simulink model "SRT_ECU_1"  (R2014a)
settings: Solver=FixedStepDiscrete  StartTime=0.0  StopTime=10.0  FixedStep=0.0005  RelTol=1e-3
libraries: ec55xxlib x10
settings Model: Creator=liuencheng  LastModifiedBy=liuencheng
settings OptimizationCC: InlineParams=on  InlineInvariantSignals=on  RollThreshold=9  StateBitsets=on  DataBitsets=on  UseTempVars=on  ZeroExternalMemoryAtStartup=off  ZeroInternalMemoryAtStartup=off  EfficientFloat2IntCast=on  OptimizeModelRefInitCode=on  LifeSpan=1
settings DebuggingCC: InheritedTsInSrcMsg=none
settings HardwareCC: ProdLargestAtomicInteger=Long  ProdLargestAtomicFloat=Double  ProdIntDivRoundTo=Zero  ProdEndianess=BigEndian  ProdHWDeviceType=Freescale MPC5500
settings RTWCC: SystemTargetFile=ec55xx.tlc  MakeCommand=make_rtw optimized_fixed_point=1  GenerateMakefile=off  TemplateMakefile=ec55xx_lcc.tmf  Description=Target for EC55XX  GenerateReport=on  ProcessScript=ec55xx_make_rtw_hook  IncludeHyperlinkInReport=on  LaunchReport=on
settings CodeAppCC: IgnoreCustomStorageClasses=off
settings STFCustomTargetCC: ModelReferenceCompliant=off  ConcurrentExecutionCompliant=off  IncludeMdlTerminateFcn=off  GeneratePreprocessorConditionals=Use local settings  CombineOutputUpdateFcns=on  SuppressErrorStatus=on  ERTCustomFileBanners=on  SupportContinuousTime=off  SupportNonInlinedSFcns=off  MATLABClassNameForMDSCustomization=Simulink.SoftwareTarget.ERTCustomization  GRTInterface=off  SystemTargetFile=ec55xx.tlc
settings ERTTargetCC: GenerateSampleERTMain=off  ModelReferenceCompliant=off  IncludeMdlTerminateFcn=off  SuppressErrorStatus=on  GenerateASAP2=on  ERTSrcFileBannerTemplate=ec55xx_code_template.cgt  ERTHdrFileBannerTemplate=ec55xx_code_template.cgt  ERTDataSrcFileTemplate=ec55xx_code_template.cgt  ERTDataHdrFileTemplate=ec55xx_code_template.cgt  ERTCustomFileTemplate=ec55xx_file_process.tlc

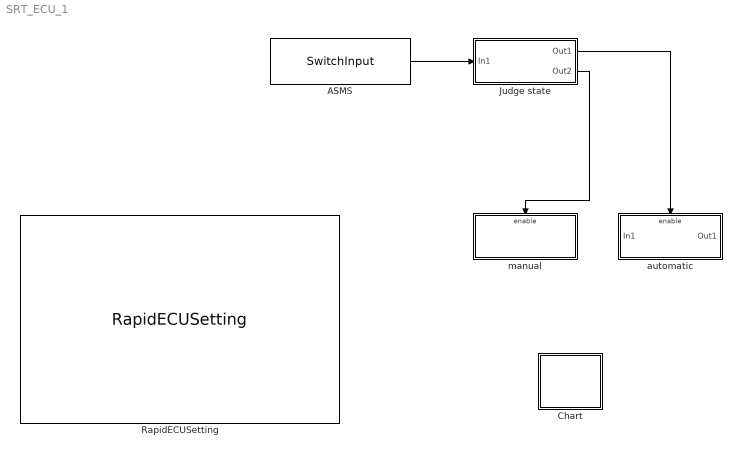
== system SRT_ECU_1 ==
  ASMS : ec55xxlib/RapidECU_U1/01SwitchInput/SwitchInput  channel=26: I_SW07_L  sampletime=-1
  Chart : Stateflow chart  TreatAsAtomicUnit=on
  Judge state : Subsystem
  RapidECUSetting : ec55xxlib/RapidECU_U2/RapidECUSetting
      link override RTI: rtiperiod=0.0005
  automatic : Subsystem  TreatAsAtomicUnit=on
  manual : Subsystem  TreatAsAtomicUnit=on
  wires:
  ASMS/1 -> Judge state/1(In1)
  Judge state/1(Out1) -> automatic/Enable
  Judge state/2(Out2) -> manual/Enable

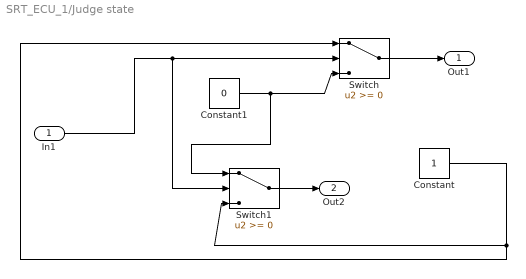
== system SRT_ECU_1/Judge state ==
  In1 : Inport
  Constant : Constant
  Constant1 : Constant  Value=0
  Switch : Switch
  Switch1 : Switch
  Out1 : Outport
  Out2 : Outport  Port=2
  wires:
  Switch/1 -> Out1/1
  Constant/1 -> Switch/1, Switch1/3
  Constant1/1 -> Switch1/1, Switch/3
  Switch1/1 -> Out2/1
  In1/1 -> Switch1/2, Switch/2

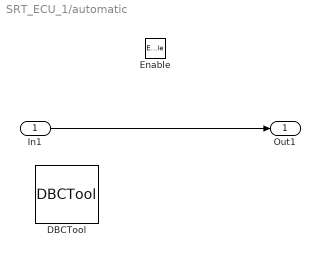
== system SRT_ECU_1/automatic ==
  In1 : Inport
  Enable : EnablePort
  DBCTool : ec55xxlib/RapidECU_U1/12DBCTool/DBCTool  dbcenable=off
  Out1 : Outport
  wires:
  In1/1 -> Out1/1

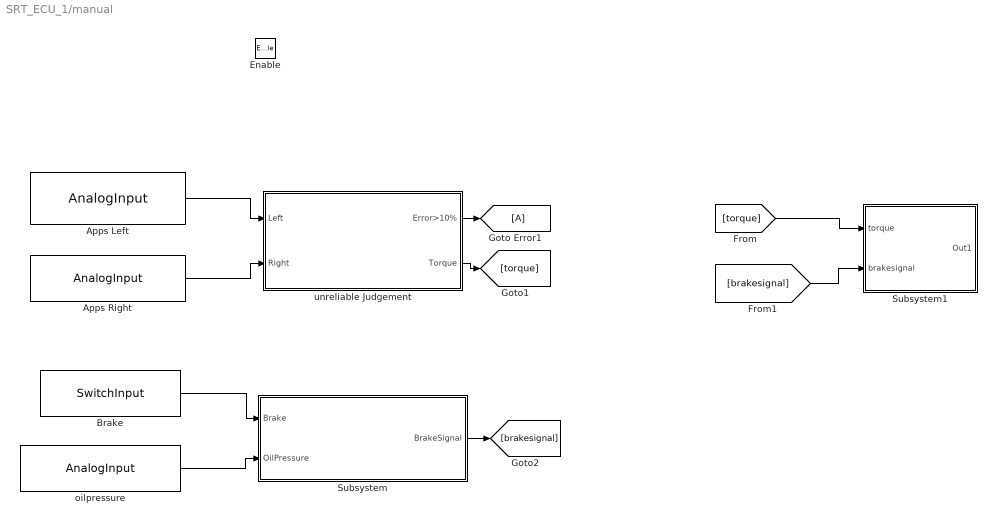
== system SRT_ECU_1/manual ==
  Enable : EnablePort
  Apps Left : ec55xxlib/RapidECU_U2/02AnalogInput/AnalogInput  channel=52: I_AN13_5V  sampletime=-1
  Apps Right : ec55xxlib/RapidECU_U2/02AnalogInput/AnalogInput  channel=53: I_AN14_5V  sampletime=-1
  "Brake " : ec55xxlib/RapidECU_U1/01SwitchInput/SwitchInput  channel=6: I_SW01_C  sampletime=-1
  Subsystem : Subsystem
  Subsystem1 : Subsystem
  "oilpressure " : ec55xxlib/RapidECU_U1/02AnalogInput/AnalogInput  channel=54: I_AN15_5V  sampletime=-1
  unreliable Judgement : Subsystem
  wires:
  Apps Left/1 -> unreliable Judgement/1(Left)
  Apps Right/1 -> unreliable Judgement/2(Right)
  unreliable Judgement/2(Torque) -> [torque]
  unreliable Judgement/1(Error>10%) -> [A]
  "Brake "/1 -> Subsystem/1("Brake ")
  "oilpressure "/1 -> Subsystem/2(OilPressure)
  Subsystem/1(BrakeSignal) -> [brakesignal]
  [torque] -> Subsystem1/1(torque)
  [brakesignal] -> Subsystem1/2(brakesignal)

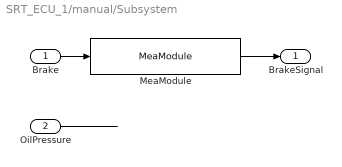
== system SRT_ECU_1/manual/Subsystem ==
  "Brake " : Inport
  OilPressure : Inport  Port=2
  MeaModule : ec55xxlib/RapidECU_U1/11Calibration/MeaModule  signal=Brake signal
  BrakeSignal : Outport
  wires:
  "Brake "/1 -> MeaModule/1
  OilPressure/1 -> ?
  MeaModule/1 -> BrakeSignal/1

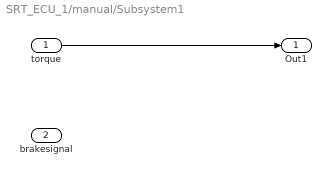
== system SRT_ECU_1/manual/Subsystem1 ==
  torque : Inport
  brakesignal : Inport  Port=2
  Out1 : Outport
  wires:
  torque/1 -> Out1/1

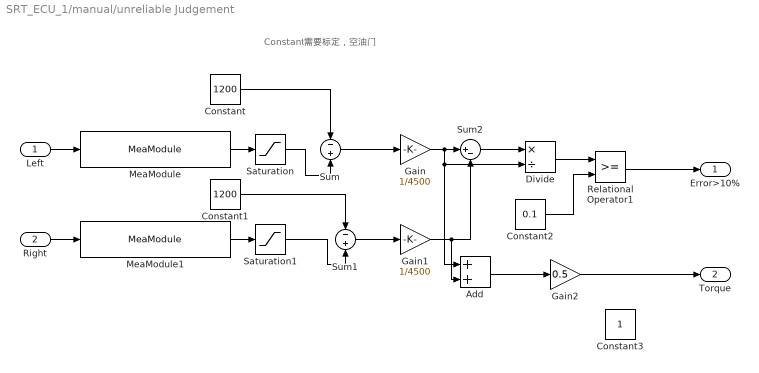
== system SRT_ECU_1/manual/unreliable Judgement ==
  note: Constant需要标定，空油门
  Left : Inport
  Right : Inport  Port=2
  Add : Sum
  Constant : Constant  Value=1200
  Constant1 : Constant  Value=1200
  Constant2 : Constant  Value=0.1
  Constant3 : Constant
  Divide : Product  Inputs=*/
  Gain : Gain  Gain=1/4500
  Gain1 : Gain  Gain=1/4500
  Gain2 : Gain  Gain=0.5
  MeaModule : ec55xxlib/RapidECU_U2/11Calibration/MeaModule  signal=Apps Left initial
  MeaModule1 : ec55xxlib/RapidECU_U2/11Calibration/MeaModule  signal=Apps Right initial
  Relational Operator1 : RelationalOperator  OutDataTypeStr=boolean
  Saturation : Saturate  UpperLimit=4500  LowerLimit=0
  Saturation1 : Saturate  UpperLimit=4500  LowerLimit=0
  Sum : Sum  Inputs=-+
  Sum1 : Sum  Inputs=-+
  Sum2 : Sum  Inputs=|+-
  Error>10% : Outport
  Torque : Outport  Port=2
  wires:
  Left/1 -> MeaModule/1
  MeaModule/1 -> Saturation/1
  Right/1 -> MeaModule1/1
  MeaModule1/1 -> Saturation1/1
  Constant/1 -> Sum/1
  Saturation/1 -> Sum/2
  Constant1/1 -> Sum1/1
  Saturation1/1 -> Sum1/2
  Sum1/1 -> Gain1/1
  Sum/1 -> Gain/1
  Gain1/1 -> Add/2, Sum2/2
  Sum2/1 -> Divide/1
  Divide/1 -> Relational Operator1/1
  Constant2/1 -> Relational Operator1/2
  Relational Operator1/1 -> Error>10%/1
  Gain/1 -> Add/1, Divide/2, Sum2/1
  Add/1 -> Gain2/1
  Gain2/1 -> Torque/1

== stateflow chart SRT_ECU_1/Chart ==
